simulink model "SensorActuator"  (R2024b)
settings: Solver=VariableStepAuto  StartTime=0  StopTime=.1  RelTol=1e-3
undefined symbols (not defined in the file or in its folder): BOOL, DINT, slplc
(part 5 of 6)

== system SensorActuator/PLC Controller Suite/__Logic/Task/Program/__Logic/XIC10/BlockEnableRead/__CoreLabelRead ==
  DataRead : DataStoreRead  DataStoreName=x_PLCLabel__s4_3653__Block_Enable  IndexOptions=Index vector (dialog)  Indices=1  OutputSizes=1
  Out1 : Outport  VectorParamsAs1DForOutWhenUnconnected=off
  wires:
  DataRead/1 -> Out1/1

== system SensorActuator/PLC Controller Suite/__Logic/Task/Program/__Logic/XIC10/Instruction_Enable/__CoreVarRead ==
  DataRead : DataStoreRead  DataStoreName=xxx_PLC_VAR_State3  IndexOptions=Index vector (dialog)  Indices=1  OutputSizes=1
  y : Outport  VectorParamsAs1DForOutWhenUnconnected=off
  wires:
  DataRead/1 -> y/1

== system SensorActuator/PLC Controller Suite/__Logic/Task/Program/__Logic/XIC10/RungInOverride/ForceRungInFalseRead ==
  __CoreLabelRead : Subsystem  Tag=CoreVarReadBlock  DisableCoverage=on  TreatAsAtomicUnit=on  mask{PLCBlockType=CoreLabelRead}
      mask init:
      | slplc.callbacks.initRoutineLabelRead(gcb);
      mask Help: web([docroot '/plccoder/ref/__corelabelread' '.html']);
      mask DialogControl PLCBlockTitle Prompt: Core Label Read
  Out1 : Outport  VectorParamsAs1DForOutWhenUnconnected=off
  wires:
  __CoreLabelRead/1(Out1) -> Out1/1

== system SensorActuator/PLC Controller Suite/__Logic/Task/Program/__Logic/XIC12/BlockEnableRead/__CoreLabelRead ==
  DataRead : DataStoreRead  DataStoreName=x_PLCLabel__s4_3653__Block_Enable  IndexOptions=Index vector (dialog)  Indices=1  OutputSizes=1
  Out1 : Outport  VectorParamsAs1DForOutWhenUnconnected=off
  wires:
  DataRead/1 -> Out1/1

== system SensorActuator/PLC Controller Suite/__Logic/Task/Program/__Logic/XIC12/Instruction_Enable/__CoreVarRead ==
  DataRead : DataStoreRead  DataStoreName=xxx_PLC_VAR_State1  IndexOptions=Index vector (dialog)  Indices=1  OutputSizes=1
  y : Outport  VectorParamsAs1DForOutWhenUnconnected=off
  wires:
  DataRead/1 -> y/1

== system SensorActuator/PLC Controller Suite/__Logic/Task/Program/__Logic/XIC12/RungInOverride/ForceRungInFalseRead ==
  __CoreLabelRead : Subsystem  Tag=CoreVarReadBlock  DisableCoverage=on  TreatAsAtomicUnit=on  mask{PLCBlockType=CoreLabelRead}
      mask init:
      | slplc.callbacks.initRoutineLabelRead(gcb);
      mask Help: web([docroot '/plccoder/ref/__corelabelread' '.html']);
      mask DialogControl PLCBlockTitle Prompt: Core Label Read
  Out1 : Outport  VectorParamsAs1DForOutWhenUnconnected=off
  wires:
  __CoreLabelRead/1(Out1) -> Out1/1

== system SensorActuator/PLC Controller Suite/__Logic/Task/Program/__Logic/XIC13/BlockEnableRead/__CoreLabelRead ==
  DataRead : DataStoreRead  DataStoreName=x_PLCLabel__s4_3653__Block_Enable  IndexOptions=Index vector (dialog)  Indices=1  OutputSizes=1
  Out1 : Outport  VectorParamsAs1DForOutWhenUnconnected=off
  wires:
  DataRead/1 -> Out1/1

== system SensorActuator/PLC Controller Suite/__Logic/Task/Program/__Logic/XIC13/Instruction_Enable/__CoreVarRead ==
  DataRead : DataStoreRead  DataStoreName=xxx_PLC_VAR_State2  IndexOptions=Index vector (dialog)  Indices=1  OutputSizes=1
  y : Outport  VectorParamsAs1DForOutWhenUnconnected=off
  wires:
  DataRead/1 -> y/1

== system SensorActuator/PLC Controller Suite/__Logic/Task/Program/__Logic/XIC13/RungInOverride/ForceRungInFalseRead ==
  __CoreLabelRead : Subsystem  Tag=CoreVarReadBlock  DisableCoverage=on  TreatAsAtomicUnit=on  mask{PLCBlockType=CoreLabelRead}
      mask init:
      | slplc.callbacks.initRoutineLabelRead(gcb);
      mask Help: web([docroot '/plccoder/ref/__corelabelread' '.html']);
      mask DialogControl PLCBlockTitle Prompt: Core Label Read
  Out1 : Outport  VectorParamsAs1DForOutWhenUnconnected=off
  wires:
  __CoreLabelRead/1(Out1) -> Out1/1

== system SensorActuator/PLC Controller Suite/__Logic/Task/Program/__Logic/XIC14/BlockEnableRead/__CoreLabelRead ==
  DataRead : DataStoreRead  DataStoreName=x_PLCLabel__s4_3653__Block_Enable  IndexOptions=Index vector (dialog)  Indices=1  OutputSizes=1
  Out1 : Outport  VectorParamsAs1DForOutWhenUnconnected=off
  wires:
  DataRead/1 -> Out1/1

== system SensorActuator/PLC Controller Suite/__Logic/Task/Program/__Logic/XIC14/Instruction_Enable/__CoreVarRead ==
  DataRead : DataStoreRead  DataStoreName=xxx_PLC_VAR_State2  IndexOptions=Index vector (dialog)  Indices=1  OutputSizes=1
  y : Outport  VectorParamsAs1DForOutWhenUnconnected=off
  wires:
  DataRead/1 -> y/1

== system SensorActuator/PLC Controller Suite/__Logic/Task/Program/__Logic/XIC14/RungInOverride/ForceRungInFalseRead ==
  __CoreLabelRead : Subsystem  Tag=CoreVarReadBlock  DisableCoverage=on  TreatAsAtomicUnit=on  mask{PLCBlockType=CoreLabelRead}
      mask init:
      | slplc.callbacks.initRoutineLabelRead(gcb);
      mask Help: web([docroot '/plccoder/ref/__corelabelread' '.html']);
      mask DialogControl PLCBlockTitle Prompt: Core Label Read
  Out1 : Outport  VectorParamsAs1DForOutWhenUnconnected=off
  wires:
  __CoreLabelRead/1(Out1) -> Out1/1

== system SensorActuator/PLC Controller Suite/__Logic/Task/Program/__Logic/XIC15/BlockEnableRead/__CoreLabelRead ==
  DataRead : DataStoreRead  DataStoreName=x_PLCLabel__s4_3653__Block_Enable  IndexOptions=Index vector (dialog)  Indices=1  OutputSizes=1
  Out1 : Outport  VectorParamsAs1DForOutWhenUnconnected=off
  wires:
  DataRead/1 -> Out1/1

== system SensorActuator/PLC Controller Suite/__Logic/Task/Program/__Logic/XIC15/Instruction_Enable/__CoreVarRead ==
  DataRead : DataStoreRead  DataStoreName=xxx_PLC_VAR_State3  IndexOptions=Index vector (dialog)  Indices=1  OutputSizes=1
  y : Outport  VectorParamsAs1DForOutWhenUnconnected=off
  wires:
  DataRead/1 -> y/1

== system SensorActuator/PLC Controller Suite/__Logic/Task/Program/__Logic/XIC15/RungInOverride/ForceRungInFalseRead ==
  __CoreLabelRead : Subsystem  Tag=CoreVarReadBlock  DisableCoverage=on  TreatAsAtomicUnit=on  mask{PLCBlockType=CoreLabelRead}
      mask init:
      | slplc.callbacks.initRoutineLabelRead(gcb);
      mask Help: web([docroot '/plccoder/ref/__corelabelread' '.html']);
      mask DialogControl PLCBlockTitle Prompt: Core Label Read
  Out1 : Outport  VectorParamsAs1DForOutWhenUnconnected=off
  wires:
  __CoreLabelRead/1(Out1) -> Out1/1

== system SensorActuator/PLC Controller Suite/__Logic/Task/Program/__Logic/XIC2/BlockEnableRead/__CoreLabelRead ==
  DataRead : DataStoreRead  DataStoreName=x_PLCLabel__s4_3653__Block_Enable  IndexOptions=Index vector (dialog)  Indices=1  OutputSizes=1
  Out1 : Outport  VectorParamsAs1DForOutWhenUnconnected=off
  wires:
  DataRead/1 -> Out1/1

== system SensorActuator/PLC Controller Suite/__Logic/Task/Program/__Logic/XIC2/Instruction_Enable/__CoreVarRead ==
  DataRead : DataStoreRead  DataStoreName=xxx_PLC_VAR_State1  IndexOptions=Index vector (dialog)  Indices=1  OutputSizes=1
  y : Outport  VectorParamsAs1DForOutWhenUnconnected=off
  wires:
  DataRead/1 -> y/1

== system SensorActuator/PLC Controller Suite/__Logic/Task/Program/__Logic/XIC2/RungInOverride/ForceRungInFalseRead ==
  __CoreLabelRead : Subsystem  Tag=CoreVarReadBlock  DisableCoverage=on  TreatAsAtomicUnit=on  mask{PLCBlockType=CoreLabelRead}
      mask init:
      | slplc.callbacks.initRoutineLabelRead(gcb);
      mask Help: web([docroot '/plccoder/ref/__corelabelread' '.html']);
      mask DialogControl PLCBlockTitle Prompt: Core Label Read
  Out1 : Outport  VectorParamsAs1DForOutWhenUnconnected=off
  wires:
  __CoreLabelRead/1(Out1) -> Out1/1

== system SensorActuator/PLC Controller Suite/__Logic/Task/Program/__Logic/XIC4/BlockEnableRead/__CoreLabelRead ==
  DataRead : DataStoreRead  DataStoreName=x_PLCLabel__s4_3653__Block_Enable  IndexOptions=Index vector (dialog)  Indices=1  OutputSizes=1
  Out1 : Outport  VectorParamsAs1DForOutWhenUnconnected=off
  wires:
  DataRead/1 -> Out1/1

== system SensorActuator/PLC Controller Suite/__Logic/Task/Program/__Logic/XIC4/Instruction_Enable/__CoreVarRead ==
  DataRead : DataStoreRead  DataStoreName=xxx_PLC_VAR_State1  IndexOptions=Index vector (dialog)  Indices=1  OutputSizes=1
  y : Outport  VectorParamsAs1DForOutWhenUnconnected=off
  wires:
  DataRead/1 -> y/1

== system SensorActuator/PLC Controller Suite/__Logic/Task/Program/__Logic/XIC4/RungInOverride/ForceRungInFalseRead ==
  __CoreLabelRead : Subsystem  Tag=CoreVarReadBlock  DisableCoverage=on  TreatAsAtomicUnit=on  mask{PLCBlockType=CoreLabelRead}
      mask init:
      | slplc.callbacks.initRoutineLabelRead(gcb);
      mask Help: web([docroot '/plccoder/ref/__corelabelread' '.html']);
      mask DialogControl PLCBlockTitle Prompt: Core Label Read
  Out1 : Outport  VectorParamsAs1DForOutWhenUnconnected=off
  wires:
  __CoreLabelRead/1(Out1) -> Out1/1

== system SensorActuator/PLC Controller Suite/__Logic/Task/Program/__Logic/XIC5/BlockEnableRead/__CoreLabelRead ==
  DataRead : DataStoreRead  DataStoreName=x_PLCLabel__s4_3653__Block_Enable  IndexOptions=Index vector (dialog)  Indices=1  OutputSizes=1
  Out1 : Outport  VectorParamsAs1DForOutWhenUnconnected=off
  wires:
  DataRead/1 -> Out1/1

== system SensorActuator/PLC Controller Suite/__Logic/Task/Program/__Logic/XIC5/Instruction_Enable/__CoreVarRead ==
  DataRead : DataStoreRead  DataStoreName=xxx_PLC_VAR_Sensor  IndexOptions=Index vector (dialog)  Indices=1  OutputSizes=1
  y : Outport  VectorParamsAs1DForOutWhenUnconnected=off
  wires:
  DataRead/1 -> y/1

== system SensorActuator/PLC Controller Suite/__Logic/Task/Program/__Logic/XIC5/RungInOverride/ForceRungInFalseRead ==
  __CoreLabelRead : Subsystem  Tag=CoreVarReadBlock  DisableCoverage=on  TreatAsAtomicUnit=on  mask{PLCBlockType=CoreLabelRead}
      mask init:
      | slplc.callbacks.initRoutineLabelRead(gcb);
      mask Help: web([docroot '/plccoder/ref/__corelabelread' '.html']);
      mask DialogControl PLCBlockTitle Prompt: Core Label Read
  Out1 : Outport  VectorParamsAs1DForOutWhenUnconnected=off
  wires:
  __CoreLabelRead/1(Out1) -> Out1/1

== system SensorActuator/PLC Controller Suite/__Logic/Task/Program/__Logic/XIC6/BlockEnableRead/__CoreLabelRead ==
  DataRead : DataStoreRead  DataStoreName=x_PLCLabel__s4_3653__Block_Enable  IndexOptions=Index vector (dialog)  Indices=1  OutputSizes=1
  Out1 : Outport  VectorParamsAs1DForOutWhenUnconnected=off
  wires:
  DataRead/1 -> Out1/1

== system SensorActuator/PLC Controller Suite/__Logic/Task/Program/__Logic/XIC6/Instruction_Enable/__CoreVarRead ==
  DataRead : DataStoreRead  DataStoreName=xxx_PLC_VAR_State2  IndexOptions=Index vector (dialog)  Indices=1  OutputSizes=1
  y : Outport  VectorParamsAs1DForOutWhenUnconnected=off
  wires:
  DataRead/1 -> y/1

== system SensorActuator/PLC Controller Suite/__Logic/Task/Program/__Logic/XIC6/RungInOverride/ForceRungInFalseRead ==
  __CoreLabelRead : Subsystem  Tag=CoreVarReadBlock  DisableCoverage=on  TreatAsAtomicUnit=on  mask{PLCBlockType=CoreLabelRead}
      mask init:
      | slplc.callbacks.initRoutineLabelRead(gcb);
      mask Help: web([docroot '/plccoder/ref/__corelabelread' '.html']);
      mask DialogControl PLCBlockTitle Prompt: Core Label Read
  Out1 : Outport  VectorParamsAs1DForOutWhenUnconnected=off
  wires:
  __CoreLabelRead/1(Out1) -> Out1/1

== system SensorActuator/PLC Controller Suite/__Logic/Task/Program/__Logic/XIC8/BlockEnableRead/__CoreLabelRead ==
  DataRead : DataStoreRead  DataStoreName=x_PLCLabel__s4_3653__Block_Enable  IndexOptions=Index vector (dialog)  Indices=1  OutputSizes=1
  Out1 : Outport  VectorParamsAs1DForOutWhenUnconnected=off
  wires:
  DataRead/1 -> Out1/1

== system SensorActuator/PLC Controller Suite/__Logic/Task/Program/__Logic/XIC8/Instruction_Enable/__CoreVarRead ==
  DataRead : DataStoreRead  DataStoreName=xxx_PLC_VAR_State2  IndexOptions=Index vector (dialog)  Indices=1  OutputSizes=1
  y : Outport  VectorParamsAs1DForOutWhenUnconnected=off
  wires:
  DataRead/1 -> y/1

== system SensorActuator/PLC Controller Suite/__Logic/Task/Program/__Logic/XIC8/RungInOverride/ForceRungInFalseRead ==
  __CoreLabelRead : Subsystem  Tag=CoreVarReadBlock  DisableCoverage=on  TreatAsAtomicUnit=on  mask{PLCBlockType=CoreLabelRead}
      mask init:
      | slplc.callbacks.initRoutineLabelRead(gcb);
      mask Help: web([docroot '/plccoder/ref/__corelabelread' '.html']);
      mask DialogControl PLCBlockTitle Prompt: Core Label Read
  Out1 : Outport  VectorParamsAs1DForOutWhenUnconnected=off
  wires:
  __CoreLabelRead/1(Out1) -> Out1/1

== system SensorActuator/PLC Controller Suite/__Logic/Task/Program/__Logic/XIC9/BlockEnableRead/__CoreLabelRead ==
  DataRead : DataStoreRead  DataStoreName=x_PLCLabel__s4_3653__Block_Enable  IndexOptions=Index vector (dialog)  Indices=1  OutputSizes=1
  Out1 : Outport  VectorParamsAs1DForOutWhenUnconnected=off
  wires:
  DataRead/1 -> Out1/1

== system SensorActuator/PLC Controller Suite/__Logic/Task/Program/__Logic/XIC9/Instruction_Enable/__CoreVarRead ==
  DataRead : DataStoreRead  DataStoreName=xxx_PLC_VAR_T  DataStoreElements=xxx_PLC_VAR_T.DN  IndexOptions=Index vector (dialog)  Indices=1  OutputSizes=1
  y : Outport  VectorParamsAs1DForOutWhenUnconnected=off
  wires:
  DataRead/1 -> y/1

== system SensorActuator/PLC Controller Suite/__Logic/Task/Program/__Logic/XIC9/RungInOverride/ForceRungInFalseRead ==
  __CoreLabelRead : Subsystem  Tag=CoreVarReadBlock  DisableCoverage=on  TreatAsAtomicUnit=on  mask{PLCBlockType=CoreLabelRead}
      mask init:
      | slplc.callbacks.initRoutineLabelRead(gcb);
      mask Help: web([docroot '/plccoder/ref/__corelabelread' '.html']);
      mask DialogControl PLCBlockTitle Prompt: Core Label Read
  Out1 : Outport  VectorParamsAs1DForOutWhenUnconnected=off
  wires:
  __CoreLabelRead/1(Out1) -> Out1/1

== system SensorActuator/PLC Controller Suite/__Logic/Task/Program/__Logic/XIO/BlockEnableRead/__CoreLabelRead ==
  DataRead : DataStoreRead  DataStoreName=x_PLCLabel__s4_3653__Block_Enable  IndexOptions=Index vector (dialog)  Indices=1  OutputSizes=1
  Out1 : Outport  VectorParamsAs1DForOutWhenUnconnected=off
  wires:
  DataRead/1 -> Out1/1

== system SensorActuator/PLC Controller Suite/__Logic/Task/Program/__Logic/XIO/Instruction_Enable/__CoreVarRead ==
  DataRead : DataStoreRead  DataStoreName=xxx_PLC_VAR_State2  IndexOptions=Index vector (dialog)  Indices=1  OutputSizes=1
  y : Outport  VectorParamsAs1DForOutWhenUnconnected=off
  wires:
  DataRead/1 -> y/1

== system SensorActuator/PLC Controller Suite/__Logic/Task/Program/__Logic/XIO/RungInOverride/ForceRungInFalseRead ==
  __CoreLabelRead : Subsystem  Tag=CoreVarReadBlock  DisableCoverage=on  TreatAsAtomicUnit=on  mask{PLCBlockType=CoreLabelRead}
      mask init:
      | slplc.callbacks.initRoutineLabelRead(gcb);
      mask Help: web([docroot '/plccoder/ref/__corelabelread' '.html']);
      mask DialogControl PLCBlockTitle Prompt: Core Label Read
  Out1 : Outport  VectorParamsAs1DForOutWhenUnconnected=off
  wires:
  __CoreLabelRead/1(Out1) -> Out1/1

== system SensorActuator/PLC Controller Suite/__Logic/Task/Program/__Logic/XIO1/BlockEnableRead/__CoreLabelRead ==
  DataRead : DataStoreRead  DataStoreName=x_PLCLabel__s4_3653__Block_Enable  IndexOptions=Index vector (dialog)  Indices=1  OutputSizes=1
  Out1 : Outport  VectorParamsAs1DForOutWhenUnconnected=off
  wires:
  DataRead/1 -> Out1/1

== system SensorActuator/PLC Controller Suite/__Logic/Task/Program/__Logic/XIO1/Instruction_Enable/__CoreVarRead ==
  DataRead : DataStoreRead  DataStoreName=xxx_PLC_VAR_State3  IndexOptions=Index vector (dialog)  Indices=1  OutputSizes=1
  y : Outport  VectorParamsAs1DForOutWhenUnconnected=off
  wires:
  DataRead/1 -> y/1

== system SensorActuator/PLC Controller Suite/__Logic/Task/Program/__Logic/XIO1/RungInOverride/ForceRungInFalseRead ==
  __CoreLabelRead : Subsystem  Tag=CoreVarReadBlock  DisableCoverage=on  TreatAsAtomicUnit=on  mask{PLCBlockType=CoreLabelRead}
      mask init:
      | slplc.callbacks.initRoutineLabelRead(gcb);
      mask Help: web([docroot '/plccoder/ref/__corelabelread' '.html']);
      mask DialogControl PLCBlockTitle Prompt: Core Label Read
  Out1 : Outport  VectorParamsAs1DForOutWhenUnconnected=off
  wires:
  __CoreLabelRead/1(Out1) -> Out1/1

== system SensorActuator/PLC Controller Suite/__Logic/Task/Program/__Logic/XIO2/BlockEnableRead/__CoreLabelRead ==
  DataRead : DataStoreRead  DataStoreName=x_PLCLabel__s4_3653__Block_Enable  IndexOptions=Index vector (dialog)  Indices=1  OutputSizes=1
  Out1 : Outport  VectorParamsAs1DForOutWhenUnconnected=off
  wires:
  DataRead/1 -> Out1/1

== system SensorActuator/PLC Controller Suite/__Logic/Task/Program/__Logic/XIO2/Instruction_Enable/__CoreVarRead ==
  DataRead : DataStoreRead  DataStoreName=xxx_PLC_VAR_State4  IndexOptions=Index vector (dialog)  Indices=1  OutputSizes=1
  y : Outport  VectorParamsAs1DForOutWhenUnconnected=off
  wires:
  DataRead/1 -> y/1

== system SensorActuator/PLC Controller Suite/__Logic/Task/Program/__Logic/XIO2/RungInOverride/ForceRungInFalseRead ==
  __CoreLabelRead : Subsystem  Tag=CoreVarReadBlock  DisableCoverage=on  TreatAsAtomicUnit=on  mask{PLCBlockType=CoreLabelRead}
      mask init:
      | slplc.callbacks.initRoutineLabelRead(gcb);
      mask Help: web([docroot '/plccoder/ref/__corelabelread' '.html']);
      mask DialogControl PLCBlockTitle Prompt: Core Label Read
  Out1 : Outport  VectorParamsAs1DForOutWhenUnconnected=off
  wires:
  __CoreLabelRead/1(Out1) -> Out1/1

== system SensorActuator/PLC Controller Suite/__Logic/Task/Program/__Logic/XIO3/BlockEnableRead/__CoreLabelRead ==
  DataRead : DataStoreRead  DataStoreName=x_PLCLabel__s4_3653__Block_Enable  IndexOptions=Index vector (dialog)  Indices=1  OutputSizes=1
  Out1 : Outport  VectorParamsAs1DForOutWhenUnconnected=off
  wires:
  DataRead/1 -> Out1/1

== system SensorActuator/PLC Controller Suite/__Logic/Task/Program/__Logic/XIO3/Instruction_Enable/__CoreVarRead ==
  DataRead : DataStoreRead  DataStoreName=xxx_PLC_VAR_State1  IndexOptions=Index vector (dialog)  Indices=1  OutputSizes=1
  y : Outport  VectorParamsAs1DForOutWhenUnconnected=off
  wires:
  DataRead/1 -> y/1

== system SensorActuator/PLC Controller Suite/__Logic/Task/Program/__Logic/XIO3/RungInOverride/ForceRungInFalseRead ==
  __CoreLabelRead : Subsystem  Tag=CoreVarReadBlock  DisableCoverage=on  TreatAsAtomicUnit=on  mask{PLCBlockType=CoreLabelRead}
      mask init:
      | slplc.callbacks.initRoutineLabelRead(gcb);
      mask Help: web([docroot '/plccoder/ref/__corelabelread' '.html']);
      mask DialogControl PLCBlockTitle Prompt: Core Label Read
  Out1 : Outport  VectorParamsAs1DForOutWhenUnconnected=off
  wires:
  __CoreLabelRead/1(Out1) -> Out1/1

== system SensorActuator/PLC Controller Suite/__Logic/Task/Program/__Logic/XIO4/BlockEnableRead/__CoreLabelRead ==
  DataRead : DataStoreRead  DataStoreName=x_PLCLabel__s4_3653__Block_Enable  IndexOptions=Index vector (dialog)  Indices=1  OutputSizes=1
  Out1 : Outport  VectorParamsAs1DForOutWhenUnconnected=off
  wires:
  DataRead/1 -> Out1/1

== system SensorActuator/PLC Controller Suite/__Logic/Task/Program/__Logic/XIO4/Instruction_Enable/__CoreVarRead ==
  DataRead : DataStoreRead  DataStoreName=xxx_PLC_VAR_State2  IndexOptions=Index vector (dialog)  Indices=1  OutputSizes=1
  y : Outport  VectorParamsAs1DForOutWhenUnconnected=off
  wires:
  DataRead/1 -> y/1

== system SensorActuator/PLC Controller Suite/__Logic/Task/Program/__Logic/XIO4/RungInOverride/ForceRungInFalseRead ==
  __CoreLabelRead : Subsystem  Tag=CoreVarReadBlock  DisableCoverage=on  TreatAsAtomicUnit=on  mask{PLCBlockType=CoreLabelRead}
      mask init:
      | slplc.callbacks.initRoutineLabelRead(gcb);
      mask Help: web([docroot '/plccoder/ref/__corelabelread' '.html']);
      mask DialogControl PLCBlockTitle Prompt: Core Label Read
  Out1 : Outport  VectorParamsAs1DForOutWhenUnconnected=off
  wires:
  __CoreLabelRead/1(Out1) -> Out1/1

== system SensorActuator/PLC Controller Suite/__Logic/Task/Program/__Logic/XIO5/BlockEnableRead/__CoreLabelRead ==
  DataRead : DataStoreRead  DataStoreName=x_PLCLabel__s4_3653__Block_Enable  IndexOptions=Index vector (dialog)  Indices=1  OutputSizes=1
  Out1 : Outport  VectorParamsAs1DForOutWhenUnconnected=off
  wires:
  DataRead/1 -> Out1/1

== system SensorActuator/PLC Controller Suite/__Logic/Task/Program/__Logic/XIO5/Instruction_Enable/__CoreVarRead ==
  DataRead : DataStoreRead  DataStoreName=xxx_PLC_VAR_State3  IndexOptions=Index vector (dialog)  Indices=1  OutputSizes=1
  y : Outport  VectorParamsAs1DForOutWhenUnconnected=off
  wires:
  DataRead/1 -> y/1

== system SensorActuator/PLC Controller Suite/__Logic/Task/Program/__Logic/XIO5/RungInOverride/ForceRungInFalseRead ==
  __CoreLabelRead : Subsystem  Tag=CoreVarReadBlock  DisableCoverage=on  TreatAsAtomicUnit=on  mask{PLCBlockType=CoreLabelRead}
      mask init:
      | slplc.callbacks.initRoutineLabelRead(gcb);
      mask Help: web([docroot '/plccoder/ref/__corelabelread' '.html']);
      mask DialogControl PLCBlockTitle Prompt: Core Label Read
  Out1 : Outport  VectorParamsAs1DForOutWhenUnconnected=off
  wires:
  __CoreLabelRead/1(Out1) -> Out1/1

== system SensorActuator/PLC Controller Suite/__Logic/Task/Program/__Logic/XIO6/BlockEnableRead/__CoreLabelRead ==
  DataRead : DataStoreRead  DataStoreName=x_PLCLabel__s4_3653__Block_Enable  IndexOptions=Index vector (dialog)  Indices=1  OutputSizes=1
  Out1 : Outport  VectorParamsAs1DForOutWhenUnconnected=off
  wires:
  DataRead/1 -> Out1/1

== system SensorActuator/PLC Controller Suite/__Logic/Task/Program/__Logic/XIO6/Instruction_Enable/__CoreVarRead ==
  DataRead : DataStoreRead  DataStoreName=xxx_PLC_VAR_State4  IndexOptions=Index vector (dialog)  Indices=1  OutputSizes=1
  y : Outport  VectorParamsAs1DForOutWhenUnconnected=off
  wires:
  DataRead/1 -> y/1

== system SensorActuator/PLC Controller Suite/__Logic/Task/Program/__Logic/XIO6/RungInOverride/ForceRungInFalseRead ==
  __CoreLabelRead : Subsystem  Tag=CoreVarReadBlock  DisableCoverage=on  TreatAsAtomicUnit=on  mask{PLCBlockType=CoreLabelRead}
      mask init:
      | slplc.callbacks.initRoutineLabelRead(gcb);
      mask Help: web([docroot '/plccoder/ref/__corelabelread' '.html']);
      mask DialogControl PLCBlockTitle Prompt: Core Label Read
  Out1 : Outport  VectorParamsAs1DForOutWhenUnconnected=off
  wires:
  __CoreLabelRead/1(Out1) -> Out1/1

== system SensorActuator/PLC Controller Suite/__Logic/Task/Program/__Logic/OTE/Instruction_Enable/Initialize Function/__CoreVarWrite ==
  u : Inport
  DataWrite : DataStoreWrite  DataStoreName=xxx_PLC_VAR_Motor  IndexOptions=Index vector (dialog)  Indices=1  OutputSizes=1
  wires:
  u/1 -> DataWrite/1

== system SensorActuator/PLC Controller Suite/__Logic/Task/Program/__Logic/OTE/Instruction_Enable/Rung-condition is false/__CoreVarWrite ==
  u : Inport
  DataWrite : DataStoreWrite  DataStoreName=xxx_PLC_VAR_Motor  IndexOptions=Index vector (dialog)  Indices=1  OutputSizes=1
  wires:
  u/1 -> DataWrite/1

== system SensorActuator/PLC Controller Suite/__Logic/Task/Program/__Logic/OTE/Instruction_Enable/Rung-condition-in is true/__CoreVarWrite ==
  u : Inport
  DataWrite : DataStoreWrite  DataStoreName=xxx_PLC_VAR_Motor  IndexOptions=Index vector (dialog)  Indices=1  OutputSizes=1
  wires:
  u/1 -> DataWrite/1

== system SensorActuator/PLC Controller Suite/__Logic/Task/Program/__Logic/OTE/RungInOverride/ForceRungInFalseRead/__CoreLabelRead ==
  DataRead : DataStoreRead  DataStoreName=x_PLCLabel__s4_3653__Force_RungIn_False  IndexOptions=Index vector (dialog)  Indices=1  OutputSizes=1
  Out1 : Outport  VectorParamsAs1DForOutWhenUnconnected=off
  wires:
  DataRead/1 -> Out1/1

== system SensorActuator/PLC Controller Suite/__Logic/Task/Program/__Logic/OTE1/Instruction_Enable/Initialize Function/__CoreVarWrite ==
  u : Inport
  DataWrite : DataStoreWrite  DataStoreName=xxx_PLC_VAR_Actuator  IndexOptions=Index vector (dialog)  Indices=1  OutputSizes=1
  wires:
  u/1 -> DataWrite/1

== system SensorActuator/PLC Controller Suite/__Logic/Task/Program/__Logic/OTE1/Instruction_Enable/Rung-condition is false/__CoreVarWrite ==
  u : Inport
  DataWrite : DataStoreWrite  DataStoreName=xxx_PLC_VAR_Actuator  IndexOptions=Index vector (dialog)  Indices=1  OutputSizes=1
  wires:
  u/1 -> DataWrite/1

== system SensorActuator/PLC Controller Suite/__Logic/Task/Program/__Logic/OTE1/Instruction_Enable/Rung-condition-in is true/__CoreVarWrite ==
  u : Inport
  DataWrite : DataStoreWrite  DataStoreName=xxx_PLC_VAR_Actuator  IndexOptions=Index vector (dialog)  Indices=1  OutputSizes=1
  wires:
  u/1 -> DataWrite/1

== system SensorActuator/PLC Controller Suite/__Logic/Task/Program/__Logic/OTE1/RungInOverride/ForceRungInFalseRead/__CoreLabelRead ==
  DataRead : DataStoreRead  DataStoreName=x_PLCLabel__s4_3653__Force_RungIn_False  IndexOptions=Index vector (dialog)  Indices=1  OutputSizes=1
  Out1 : Outport  VectorParamsAs1DForOutWhenUnconnected=off
  wires:
  DataRead/1 -> Out1/1

== system SensorActuator/PLC Controller Suite/__Logic/Task/Program/__Logic/OTE2/Instruction_Enable/Initialize Function/__CoreVarWrite ==
  u : Inport
  DataWrite : DataStoreWrite  DataStoreName=xxx_PLC_VAR_State0  IndexOptions=Index vector (dialog)  Indices=1  OutputSizes=1
  wires:
  u/1 -> DataWrite/1

== system SensorActuator/PLC Controller Suite/__Logic/Task/Program/__Logic/OTE2/Instruction_Enable/Rung-condition is false/__CoreVarWrite ==
  u : Inport
  DataWrite : DataStoreWrite  DataStoreName=xxx_PLC_VAR_State0  IndexOptions=Index vector (dialog)  Indices=1  OutputSizes=1
  wires:
  u/1 -> DataWrite/1

== system SensorActuator/PLC Controller Suite/__Logic/Task/Program/__Logic/OTE2/Instruction_Enable/Rung-condition-in is true/__CoreVarWrite ==
  u : Inport
  DataWrite : DataStoreWrite  DataStoreName=xxx_PLC_VAR_State0  IndexOptions=Index vector (dialog)  Indices=1  OutputSizes=1
  wires:
  u/1 -> DataWrite/1

== system SensorActuator/PLC Controller Suite/__Logic/Task/Program/__Logic/OTE2/RungInOverride/ForceRungInFalseRead/__CoreLabelRead ==
  DataRead : DataStoreRead  DataStoreName=x_PLCLabel__s4_3653__Force_RungIn_False  IndexOptions=Index vector (dialog)  Indices=1  OutputSizes=1
  Out1 : Outport  VectorParamsAs1DForOutWhenUnconnected=off
  wires:
  DataRead/1 -> Out1/1

== system SensorActuator/PLC Controller Suite/__Logic/Task/Program/__Logic/OTE3/Instruction_Enable/Initialize Function/__CoreVarWrite ==
  u : Inport
  DataWrite : DataStoreWrite  DataStoreName=xxx_PLC_VAR_State1  IndexOptions=Index vector (dialog)  Indices=1  OutputSizes=1
  wires:
  u/1 -> DataWrite/1

== system SensorActuator/PLC Controller Suite/__Logic/Task/Program/__Logic/OTE3/Instruction_Enable/Rung-condition is false/__CoreVarWrite ==
  u : Inport
  DataWrite : DataStoreWrite  DataStoreName=xxx_PLC_VAR_State1  IndexOptions=Index vector (dialog)  Indices=1  OutputSizes=1
  wires:
  u/1 -> DataWrite/1

== system SensorActuator/PLC Controller Suite/__Logic/Task/Program/__Logic/OTE3/Instruction_Enable/Rung-condition-in is true/__CoreVarWrite ==
  u : Inport
  DataWrite : DataStoreWrite  DataStoreName=xxx_PLC_VAR_State1  IndexOptions=Index vector (dialog)  Indices=1  OutputSizes=1
  wires:
  u/1 -> DataWrite/1

== system SensorActuator/PLC Controller Suite/__Logic/Task/Program/__Logic/OTE3/RungInOverride/ForceRungInFalseRead/__CoreLabelRead ==
  DataRead : DataStoreRead  DataStoreName=x_PLCLabel__s4_3653__Force_RungIn_False  IndexOptions=Index vector (dialog)  Indices=1  OutputSizes=1
  Out1 : Outport  VectorParamsAs1DForOutWhenUnconnected=off
  wires:
  DataRead/1 -> Out1/1

== system SensorActuator/PLC Controller Suite/__Logic/Task/Program/__Logic/OTE4/Instruction_Enable/Initialize Function/__CoreVarWrite ==
  u : Inport
  DataWrite : DataStoreWrite  DataStoreName=xxx_PLC_VAR_State2  IndexOptions=Index vector (dialog)  Indices=1  OutputSizes=1
  wires:
  u/1 -> DataWrite/1

== system SensorActuator/PLC Controller Suite/__Logic/Task/Program/__Logic/OTE4/Instruction_Enable/Rung-condition is false/__CoreVarWrite ==
  u : Inport
  DataWrite : DataStoreWrite  DataStoreName=xxx_PLC_VAR_State2  IndexOptions=Index vector (dialog)  Indices=1  OutputSizes=1
  wires:
  u/1 -> DataWrite/1

== system SensorActuator/PLC Controller Suite/__Logic/Task/Program/__Logic/OTE4/Instruction_Enable/Rung-condition-in is true/__CoreVarWrite ==
  u : Inport
  DataWrite : DataStoreWrite  DataStoreName=xxx_PLC_VAR_State2  IndexOptions=Index vector (dialog)  Indices=1  OutputSizes=1
  wires:
  u/1 -> DataWrite/1

== system SensorActuator/PLC Controller Suite/__Logic/Task/Program/__Logic/OTE4/RungInOverride/ForceRungInFalseRead/__CoreLabelRead ==
  DataRead : DataStoreRead  DataStoreName=x_PLCLabel__s4_3653__Force_RungIn_False  IndexOptions=Index vector (dialog)  Indices=1  OutputSizes=1
  Out1 : Outport  VectorParamsAs1DForOutWhenUnconnected=off
  wires:
  DataRead/1 -> Out1/1

== system SensorActuator/PLC Controller Suite/__Logic/Task/Program/__Logic/OTE5/Instruction_Enable/Initialize Function/__CoreVarWrite ==
  u : Inport
  DataWrite : DataStoreWrite  DataStoreName=xxx_PLC_VAR_State3  IndexOptions=Index vector (dialog)  Indices=1  OutputSizes=1
  wires:
  u/1 -> DataWrite/1

== system SensorActuator/PLC Controller Suite/__Logic/Task/Program/__Logic/OTE5/Instruction_Enable/Rung-condition is false/__CoreVarWrite ==
  u : Inport
  DataWrite : DataStoreWrite  DataStoreName=xxx_PLC_VAR_State3  IndexOptions=Index vector (dialog)  Indices=1  OutputSizes=1
  wires:
  u/1 -> DataWrite/1

== system SensorActuator/PLC Controller Suite/__Logic/Task/Program/__Logic/OTE5/Instruction_Enable/Rung-condition-in is true/__CoreVarWrite ==
  u : Inport
  DataWrite : DataStoreWrite  DataStoreName=xxx_PLC_VAR_State3  IndexOptions=Index vector (dialog)  Indices=1  OutputSizes=1
  wires:
  u/1 -> DataWrite/1

== system SensorActuator/PLC Controller Suite/__Logic/Task/Program/__Logic/OTE5/RungInOverride/ForceRungInFalseRead/__CoreLabelRead ==
  DataRead : DataStoreRead  DataStoreName=x_PLCLabel__s4_3653__Force_RungIn_False  IndexOptions=Index vector (dialog)  Indices=1  OutputSizes=1
  Out1 : Outport  VectorParamsAs1DForOutWhenUnconnected=off
  wires:
  DataRead/1 -> Out1/1

== system SensorActuator/PLC Controller Suite/__Logic/Task/Program/__Logic/TON/Instruction_Enable/Initialize Function/VarWrite ==
  In1 : Inport
  __CoreVarWrite : Subsystem  Tag=CoreVarWriteBlock  DisableCoverage=on  TreatAsAtomicUnit=on  mask{PLCBlockType=CoreVarWrite}
      mask init:
      | slplc.callbacks.initCoreVariable(gcb, 'write');
      mask Help: web([docroot '/plccoder/ref/__corevarwrite' '.html']);
      mask DialogControl PLCBlockTitle Prompt: Core Variable Write
  wires:
  In1/1 -> __CoreVarWrite/1(u)

== system SensorActuator/PLC Controller Suite/__Logic/Task/Program/__Logic/TON/Instruction_Enable/Initialize Function/VarWrite1 ==
  In1 : Inport
  __CoreVarWrite : Subsystem  Tag=CoreVarWriteBlock  DisableCoverage=on  TreatAsAtomicUnit=on  mask{PLCBlockType=CoreVarWrite}
      mask init:
      | slplc.callbacks.initCoreVariable(gcb, 'write');
      mask Help: web([docroot '/plccoder/ref/__corevarwrite' '.html']);
      mask DialogControl PLCBlockTitle Prompt: Core Variable Write
  wires:
  In1/1 -> __CoreVarWrite/1(u)

== system SensorActuator/PLC Controller Suite/__Logic/Task/Program/__Logic/TON/Instruction_Enable/Initialize Function/VarWrite2 ==
  In1 : Inport
  __CoreVarWrite : Subsystem  Tag=CoreVarWriteBlock  DisableCoverage=on  TreatAsAtomicUnit=on  mask{PLCBlockType=CoreVarWrite}
      mask init:
      | slplc.callbacks.initCoreVariable(gcb, 'write');
      mask Help: web([docroot '/plccoder/ref/__corevarwrite' '.html']);
      mask DialogControl PLCBlockTitle Prompt: Core Variable Write
  wires:
  In1/1 -> __CoreVarWrite/1(u)

== system SensorActuator/PLC Controller Suite/__Logic/Task/Program/__Logic/TON/Instruction_Enable/Initialize Function/VarWrite3 ==
  In1 : Inport
  __CoreVarWrite : Subsystem  Tag=CoreVarWriteBlock  DisableCoverage=on  TreatAsAtomicUnit=on  mask{PLCBlockType=CoreVarWrite}
      mask init:
      | slplc.callbacks.initCoreVariable(gcb, 'write');
      mask Help: web([docroot '/plccoder/ref/__corevarwrite' '.html']);
      mask DialogControl PLCBlockTitle Prompt: Core Variable Write
  wires:
  In1/1 -> __CoreVarWrite/1(u)

== system SensorActuator/PLC Controller Suite/__Logic/Task/Program/__Logic/TON/RungInOverride/ForceRungInFalseRead/__CoreLabelRead ==
  DataRead : DataStoreRead  DataStoreName=x_PLCLabel__s4_3653__Force_RungIn_False  IndexOptions=Index vector (dialog)  Indices=1  OutputSizes=1
  Out1 : Outport  VectorParamsAs1DForOutWhenUnconnected=off
  wires:
  DataRead/1 -> Out1/1

== system SensorActuator/PLC Controller Suite/__Logic/Task/Program/__Logic/XIC/RungInOverride/ForceRungInFalseRead/__CoreLabelRead ==
  DataRead : DataStoreRead  DataStoreName=x_PLCLabel__s4_3653__Force_RungIn_False  IndexOptions=Index vector (dialog)  Indices=1  OutputSizes=1
  Out1 : Outport  VectorParamsAs1DForOutWhenUnconnected=off
  wires:
  DataRead/1 -> Out1/1

== system SensorActuator/PLC Controller Suite/__Logic/Task/Program/__Logic/XIC1/RungInOverride/ForceRungInFalseRead/__CoreLabelRead ==
  DataRead : DataStoreRead  DataStoreName=x_PLCLabel__s4_3653__Force_RungIn_False  IndexOptions=Index vector (dialog)  Indices=1  OutputSizes=1
  Out1 : Outport  VectorParamsAs1DForOutWhenUnconnected=off
  wires:
  DataRead/1 -> Out1/1

== system SensorActuator/PLC Controller Suite/__Logic/Task/Program/__Logic/XIC10/RungInOverride/ForceRungInFalseRead/__CoreLabelRead ==
  DataRead : DataStoreRead  DataStoreName=x_PLCLabel__s4_3653__Force_RungIn_False  IndexOptions=Index vector (dialog)  Indices=1  OutputSizes=1
  Out1 : Outport  VectorParamsAs1DForOutWhenUnconnected=off
  wires:
  DataRead/1 -> Out1/1

== system SensorActuator/PLC Controller Suite/__Logic/Task/Program/__Logic/XIC12/RungInOverride/ForceRungInFalseRead/__CoreLabelRead ==
  DataRead : DataStoreRead  DataStoreName=x_PLCLabel__s4_3653__Force_RungIn_False  IndexOptions=Index vector (dialog)  Indices=1  OutputSizes=1
  Out1 : Outport  VectorParamsAs1DForOutWhenUnconnected=off
  wires:
  DataRead/1 -> Out1/1

== system SensorActuator/PLC Controller Suite/__Logic/Task/Program/__Logic/XIC13/RungInOverride/ForceRungInFalseRead/__CoreLabelRead ==
  DataRead : DataStoreRead  DataStoreName=x_PLCLabel__s4_3653__Force_RungIn_False  IndexOptions=Index vector (dialog)  Indices=1  OutputSizes=1
  Out1 : Outport  VectorParamsAs1DForOutWhenUnconnected=off
  wires:
  DataRead/1 -> Out1/1

== system SensorActuator/PLC Controller Suite/__Logic/Task/Program/__Logic/XIC14/RungInOverride/ForceRungInFalseRead/__CoreLabelRead ==
  DataRead : DataStoreRead  DataStoreName=x_PLCLabel__s4_3653__Force_RungIn_False  IndexOptions=Index vector (dialog)  Indices=1  OutputSizes=1
  Out1 : Outport  VectorParamsAs1DForOutWhenUnconnected=off
  wires:
  DataRead/1 -> Out1/1

== system SensorActuator/PLC Controller Suite/__Logic/Task/Program/__Logic/XIC15/RungInOverride/ForceRungInFalseRead/__CoreLabelRead ==
  DataRead : DataStoreRead  DataStoreName=x_PLCLabel__s4_3653__Force_RungIn_False  IndexOptions=Index vector (dialog)  Indices=1  OutputSizes=1
  Out1 : Outport  VectorParamsAs1DForOutWhenUnconnected=off
  wires:
  DataRead/1 -> Out1/1

== system SensorActuator/PLC Controller Suite/__Logic/Task/Program/__Logic/XIC2/RungInOverride/ForceRungInFalseRead/__CoreLabelRead ==
  DataRead : DataStoreRead  DataStoreName=x_PLCLabel__s4_3653__Force_RungIn_False  IndexOptions=Index vector (dialog)  Indices=1  OutputSizes=1
  Out1 : Outport  VectorParamsAs1DForOutWhenUnconnected=off
  wires:
  DataRead/1 -> Out1/1

== system SensorActuator/PLC Controller Suite/__Logic/Task/Program/__Logic/XIC4/RungInOverride/ForceRungInFalseRead/__CoreLabelRead ==
  DataRead : DataStoreRead  DataStoreName=x_PLCLabel__s4_3653__Force_RungIn_False  IndexOptions=Index vector (dialog)  Indices=1  OutputSizes=1
  Out1 : Outport  VectorParamsAs1DForOutWhenUnconnected=off
  wires:
  DataRead/1 -> Out1/1

== system SensorActuator/PLC Controller Suite/__Logic/Task/Program/__Logic/XIC5/RungInOverride/ForceRungInFalseRead/__CoreLabelRead ==
  DataRead : DataStoreRead  DataStoreName=x_PLCLabel__s4_3653__Force_RungIn_False  IndexOptions=Index vector (dialog)  Indices=1  OutputSizes=1
  Out1 : Outport  VectorParamsAs1DForOutWhenUnconnected=off
  wires:
  DataRead/1 -> Out1/1

== system SensorActuator/PLC Controller Suite/__Logic/Task/Program/__Logic/XIC6/RungInOverride/ForceRungInFalseRead/__CoreLabelRead ==
  DataRead : DataStoreRead  DataStoreName=x_PLCLabel__s4_3653__Force_RungIn_False  IndexOptions=Index vector (dialog)  Indices=1  OutputSizes=1
  Out1 : Outport  VectorParamsAs1DForOutWhenUnconnected=off
  wires:
  DataRead/1 -> Out1/1

== system SensorActuator/PLC Controller Suite/__Logic/Task/Program/__Logic/XIC8/RungInOverride/ForceRungInFalseRead/__CoreLabelRead ==
  DataRead : DataStoreRead  DataStoreName=x_PLCLabel__s4_3653__Force_RungIn_False  IndexOptions=Index vector (dialog)  Indices=1  OutputSizes=1
  Out1 : Outport  VectorParamsAs1DForOutWhenUnconnected=off
  wires:
  DataRead/1 -> Out1/1

== system SensorActuator/PLC Controller Suite/__Logic/Task/Program/__Logic/XIC9/RungInOverride/ForceRungInFalseRead/__CoreLabelRead ==
  DataRead : DataStoreRead  DataStoreName=x_PLCLabel__s4_3653__Force_RungIn_False  IndexOptions=Index vector (dialog)  Indices=1  OutputSizes=1
  Out1 : Outport  VectorParamsAs1DForOutWhenUnconnected=off
  wires:
  DataRead/1 -> Out1/1

== system SensorActuator/PLC Controller Suite/__Logic/Task/Program/__Logic/XIO/RungInOverride/ForceRungInFalseRead/__CoreLabelRead ==
  DataRead : DataStoreRead  DataStoreName=x_PLCLabel__s4_3653__Force_RungIn_False  IndexOptions=Index vector (dialog)  Indices=1  OutputSizes=1
  Out1 : Outport  VectorParamsAs1DForOutWhenUnconnected=off
  wires:
  DataRead/1 -> Out1/1

== system SensorActuator/PLC Controller Suite/__Logic/Task/Program/__Logic/XIO1/RungInOverride/ForceRungInFalseRead/__CoreLabelRead ==
  DataRead : DataStoreRead  DataStoreName=x_PLCLabel__s4_3653__Force_RungIn_False  IndexOptions=Index vector (dialog)  Indices=1  OutputSizes=1
  Out1 : Outport  VectorParamsAs1DForOutWhenUnconnected=off
  wires:
  DataRead/1 -> Out1/1

== system SensorActuator/PLC Controller Suite/__Logic/Task/Program/__Logic/XIO2/RungInOverride/ForceRungInFalseRead/__CoreLabelRead ==
  DataRead : DataStoreRead  DataStoreName=x_PLCLabel__s4_3653__Force_RungIn_False  IndexOptions=Index vector (dialog)  Indices=1  OutputSizes=1
  Out1 : Outport  VectorParamsAs1DForOutWhenUnconnected=off
  wires:
  DataRead/1 -> Out1/1

== system SensorActuator/PLC Controller Suite/__Logic/Task/Program/__Logic/XIO3/RungInOverride/ForceRungInFalseRead/__CoreLabelRead ==
  DataRead : DataStoreRead  DataStoreName=x_PLCLabel__s4_3653__Force_RungIn_False  IndexOptions=Index vector (dialog)  Indices=1  OutputSizes=1
  Out1 : Outport  VectorParamsAs1DForOutWhenUnconnected=off
  wires:
  DataRead/1 -> Out1/1

== system SensorActuator/PLC Controller Suite/__Logic/Task/Program/__Logic/XIO4/RungInOverride/ForceRungInFalseRead/__CoreLabelRead ==
  DataRead : DataStoreRead  DataStoreName=x_PLCLabel__s4_3653__Force_RungIn_False  IndexOptions=Index vector (dialog)  Indices=1  OutputSizes=1
  Out1 : Outport  VectorParamsAs1DForOutWhenUnconnected=off
  wires:
  DataRead/1 -> Out1/1

== system SensorActuator/PLC Controller Suite/__Logic/Task/Program/__Logic/XIO5/RungInOverride/ForceRungInFalseRead/__CoreLabelRead ==
  DataRead : DataStoreRead  DataStoreName=x_PLCLabel__s4_3653__Force_RungIn_False  IndexOptions=Index vector (dialog)  Indices=1  OutputSizes=1
  Out1 : Outport  VectorParamsAs1DForOutWhenUnconnected=off
  wires:
  DataRead/1 -> Out1/1

== system SensorActuator/PLC Controller Suite/__Logic/Task/Program/__Logic/XIO6/RungInOverride/ForceRungInFalseRead/__CoreLabelRead ==
  DataRead : DataStoreRead  DataStoreName=x_PLCLabel__s4_3653__Force_RungIn_False  IndexOptions=Index vector (dialog)  Indices=1  OutputSizes=1
  Out1 : Outport  VectorParamsAs1DForOutWhenUnconnected=off
  wires:
  DataRead/1 -> Out1/1

== system SensorActuator/PLC Controller Suite/__Logic/Task/Program/__Logic/TON/Instruction_Enable/Initialize Function/VarWrite/__CoreVarWrite ==
  u : Inport
  DataWrite : DataStoreWrite  DataStoreName=xxx_PLC_VAR_T  DataStoreElements=xxx_PLC_VAR_T.ACC  IndexOptions=Index vector (dialog)  Indices=1  OutputSizes=1
  wires:
  u/1 -> DataWrite/1

== system SensorActuator/PLC Controller Suite/__Logic/Task/Program/__Logic/TON/Instruction_Enable/Initialize Function/VarWrite1/__CoreVarWrite ==
  u : Inport
  DataWrite : DataStoreWrite  DataStoreName=xxx_PLC_VAR_T  DataStoreElements=xxx_PLC_VAR_T.EN  IndexOptions=Index vector (dialog)  Indices=1  OutputSizes=1
  wires:
  u/1 -> DataWrite/1

== system SensorActuator/PLC Controller Suite/__Logic/Task/Program/__Logic/TON/Instruction_Enable/Initialize Function/VarWrite2/__CoreVarWrite ==
  u : Inport
  DataWrite : DataStoreWrite  DataStoreName=xxx_PLC_VAR_T  DataStoreElements=xxx_PLC_VAR_T.TT  IndexOptions=Index vector (dialog)  Indices=1  OutputSizes=1
  wires:
  u/1 -> DataWrite/1

== system SensorActuator/PLC Controller Suite/__Logic/Task/Program/__Logic/TON/Instruction_Enable/Initialize Function/VarWrite3/__CoreVarWrite ==
  u : Inport
  DataWrite : DataStoreWrite  DataStoreName=xxx_PLC_VAR_T  DataStoreElements=xxx_PLC_VAR_T.DN  IndexOptions=Index vector (dialog)  Indices=1  OutputSizes=1
  wires:
  u/1 -> DataWrite/1

== matlab function SensorActuator/PLC Controller Suite/__Logic/Task/Program/__Logic/OTE4/__Format ==
  data: BlockEnable input; RungIn input; RungOut input; data input
function setBlockFormat(BlockEnable, RungIn, RungOut, data)

if data~=0 && data~=1
    error('slplc:inivalidBooleanValue', 'Invalid boolean value %d', data);
end
data = logical(data);

% set parent block colors
coder.extrinsic('slplc.utils.setBlockAppearance');
persistent lastBlockEnable lastRungIn lastRungOut lastData isInit lastAnimation lastDataShow;
if isempty(lastBlockEnable)
    lastBlockEnable = true;
end
if isempty(lastRungIn)
    lastRungIn = false;
end
if isempty(lastRungOut)
    lastRungOut = false;
end
if isempty(lastData)
    lastData = data;
end
if isempty(isInit)
    isInit = true;
else
    isInit = false;
end
if isempty(lastAnimation)
    lastAnimation = false;
end
if isempty(lastDataShow)
    lastDataShow = false;
end

[animation, dataShow] = slplc.utils.setBlockAppearance('set', '%<PLCOperandTag>', {}, {}, ...
    ' = ', {'ForegroundColor'}, ...
    isInit,  ...
    BlockEnable, lastBlockEnable, ...
    RungIn,  lastRungIn, ...
    RungOut, lastRungOut, ...
    data, lastData, ...
    lastAnimation, lastDataShow);

lastBlockEnable = BlockEnable;
lastRungIn      = RungIn;
lastRungOut     = RungOut;
lastData        = data;
lastAnimation   = animation;
lastDataShow    = dataShow;
end

== matlab function SensorActuator/PLC Controller Suite/__Logic/Task/Program/__Logic/XIO1/__Format ==
  data: BlockEnable input; RungIn input; RungOut input; data input
function setBlockFormat(BlockEnable, RungIn, RungOut, data)

if data~=0 && data~=1
    error('slplc:inivalidBooleanValue', 'Invalid boolean value %d', data);
end
data = logical(data);

% set parent block colors
coder.extrinsic('slplc.utils.setBlockAppearance');
persistent lastBlockEnable lastRungIn lastRungOut lastData isInit lastAnimation lastDataShow;
if isempty(lastBlockEnable)
    lastBlockEnable = true;
end
if isempty(lastRungIn)
    lastRungIn = false;
end
if isempty(lastRungOut)
    lastRungOut = false;
end
if isempty(lastData)
    lastData = data;
end
if isempty(isInit)
    isInit = true;
else
    isInit = false;
end
if isempty(lastAnimation)
    lastAnimation = false;
end
if isempty(lastDataShow)
    lastDataShow = false;
end

[animation, dataShow] = slplc.utils.setBlockAppearance('set', '%<PLCOperandTag>', {}, {}, ...
    ' = ', {'ForegroundColor'}, ...
    isInit,  ...
    BlockEnable, lastBlockEnable, ...
    RungIn,  lastRungIn, ...
    RungOut, lastRungOut, ...
    data, lastData, ...
    lastAnimation, lastDataShow);

lastBlockEnable = BlockEnable;
lastRungIn      = RungIn;
lastRungOut     = RungOut;
lastData        = data;
lastAnimation   = animation;
lastDataShow    = dataShow;
end

== matlab function SensorActuator/PLC Controller Suite/__Logic/Task/Program/__Logic/Junction2/__Format ==
  data: BlockEnable input; RungOut input
function setBlockFormat(BlockEnable, RungOut)
% set parent block colors
coder.extrinsic('slplc.utils.setBlockAppearance');
persistent lastBlockEnable isInit lastRungOut lastAnimation lastRungOutShow;
if isempty(lastBlockEnable)
    lastBlockEnable = true;
end

if isempty(isInit)
    isInit = true;
else
    isInit = false;
end

if isempty(lastRungOut)
    lastRungOut = RungOut;
end

if isempty(lastAnimation)
    lastAnimation = false;
end

if isempty(lastRungOutShow)
    lastRungOutShow = false;
end

[animation, dataShow] = slplc.utils.setBlockAppearance('set', '', {'black', 'black'}, {}, ...
    '', {'ForegroundColor', 'BackgroundColor'}, ...
    isInit,  ...
    BlockEnable, lastBlockEnable, ...
    RungOut,   lastRungOut, ...
    RungOut,   lastRungOut, ...
    [],    [], ...
    lastAnimation, lastRungOutShow);

lastBlockEnable     = BlockEnable;
lastRungOut         = RungOut;
lastAnimation       = animation;
lastRungOutShow     = dataShow;
end

== matlab function SensorActuator/PLC Controller Suite/__Logic/Task/Program/__Logic/XIC10/__Format ==
  data: BlockEnable input; RungIn input; RungOut input; data input
function setBlockFormat(BlockEnable, RungIn, RungOut, data)

if data~=0 && data~=1
    error('slplc:inivalidBooleanValue', 'Invalid boolean value %d', data);
end
data = logical(data);

% set parent block colors
coder.extrinsic('slplc.utils.setBlockAppearance');
persistent lastBlockEnable lastRungIn lastRungOut lastData isInit lastAnimation lastDataShow;
if isempty(lastBlockEnable)
    lastBlockEnable = true;
end
if isempty(lastRungIn)
    lastRungIn = false;
end
if isempty(lastRungOut)
    lastRungOut = false;
end
if isempty(lastData)
    lastData = data;
end
if isempty(isInit)
    isInit = true;
else
    isInit = false;
end
if isempty(lastAnimation)
    lastAnimation = false;
end
if isempty(lastDataShow)
    lastDataShow = false;
end

[animation, dataShow] = slplc.utils.setBlockAppearance('set', '%<PLCOperandTag>', {}, {}, ...
    ' = ', {'ForegroundColor'}, ...
    isInit,  ...
    BlockEnable, lastBlockEnable, ...
    RungIn,  lastRungIn, ...
    RungOut, lastRungOut, ...
    data, lastData, ...
    lastAnimation, lastDataShow);

lastBlockEnable = BlockEnable;
lastRungIn      = RungIn;
lastRungOut     = RungOut;
lastData        = data;
lastAnimation   = animation;
lastDataShow    = dataShow;
end

== matlab function SensorActuator/PLC Controller Suite/__Logic/Task/Program/__Logic/OTE5/__Format ==
  data: BlockEnable input; RungIn input; RungOut input; data input
function setBlockFormat(BlockEnable, RungIn, RungOut, data)

if data~=0 && data~=1
    error('slplc:inivalidBooleanValue', 'Invalid boolean value %d', data);
end
data = logical(data);

% set parent block colors
coder.extrinsic('slplc.utils.setBlockAppearance');
persistent lastBlockEnable lastRungIn lastRungOut lastData isInit lastAnimation lastDataShow;
if isempty(lastBlockEnable)
    lastBlockEnable = true;
end
if isempty(lastRungIn)
    lastRungIn = false;
end
if isempty(lastRungOut)
    lastRungOut = false;
end
if isempty(lastData)
    lastData = data;
end
if isempty(isInit)
    isInit = true;
else
    isInit = false;
end
if isempty(lastAnimation)
    lastAnimation = false;
end
if isempty(lastDataShow)
    lastDataShow = false;
end

[animation, dataShow] = slplc.utils.setBlockAppearance('set', '%<PLCOperandTag>', {}, {}, ...
    ' = ', {'ForegroundColor'}, ...
    isInit,  ...
    BlockEnable, lastBlockEnable, ...
    RungIn,  lastRungIn, ...
    RungOut, lastRungOut, ...
    data, lastData, ...
    lastAnimation, lastDataShow);

lastBlockEnable = BlockEnable;
lastRungIn      = RungIn;
lastRungOut     = RungOut;
lastData        = data;
lastAnimation   = animation;
lastDataShow    = dataShow;
end

== matlab function SensorActuator/PLC Controller Suite/__Logic/Task/Program/__Logic/XIC8/__Format ==
  data: BlockEnable input; RungIn input; RungOut input; data input
function setBlockFormat(BlockEnable, RungIn, RungOut, data)

if data~=0 && data~=1
    error('slplc:inivalidBooleanValue', 'Invalid boolean value %d', data);
end
data = logical(data);

% set parent block colors
coder.extrinsic('slplc.utils.setBlockAppearance');
persistent lastBlockEnable lastRungIn lastRungOut lastData isInit lastAnimation lastDataShow;
if isempty(lastBlockEnable)
    lastBlockEnable = true;
end
if isempty(lastRungIn)
    lastRungIn = false;
end
if isempty(lastRungOut)
    lastRungOut = false;
end
if isempty(lastData)
    lastData = data;
end
if isempty(isInit)
    isInit = true;
else
    isInit = false;
end
if isempty(lastAnimation)
    lastAnimation = false;
end
if isempty(lastDataShow)
    lastDataShow = false;
end

[animation, dataShow] = slplc.utils.setBlockAppearance('set', '%<PLCOperandTag>', {}, {}, ...
    ' = ', {'ForegroundColor'}, ...
    isInit,  ...
    BlockEnable, lastBlockEnable, ...
    RungIn,  lastRungIn, ...
    RungOut, lastRungOut, ...
    data, lastData, ...
    lastAnimation, lastDataShow);

lastBlockEnable = BlockEnable;
lastRungIn      = RungIn;
lastRungOut     = RungOut;
lastData        = data;
lastAnimation   = animation;
lastDataShow    = dataShow;
end
